simulink model "ADC"  (R2019b)
settings: Solver=FixedStepDiscrete  StartTime=0.0  StopTime=inf  FixedStep=0.05  RelTol=1e-3
libraries: discretizing x1
settings Model: Creator=Michał  LastModifiedBy=Michał
settings OptimizationCC: DefaultParameterBehavior=Inlined  EnhancedBackFolding=on  PassReuseOutputArgsAs=Individual arguments  OptimizeBlockOrder=speed  DifferentSizesBufferReuse=on  OptimizationCustomize=off  EfficientTunableParamExpr=on
settings DebuggingCC: ParameterTunabilityLossMsg=error
settings SFSimCC: MATLABDynamicMemAlloc=off
settings RTWCC: SystemTargetFile=ert.tlc  TemplateMakefile=ert_default_tmf  GenerateReport=on  IncludeHyperlinkInReport=on  LaunchReport=on  GenerateTraceInfo=on  GenerateTraceReport=on  GenerateTraceReportSl=on  GenerateTraceReportSf=on  GenerateTraceReportEml=on
settings CodeAppCC: ForceParamTrailComments=on  IgnoreCustomStorageClasses=off  OperatorAnnotations=on  SimulinkDataObjDesc=on  SFDataObjDesc=on  InsertBlockDesc=on
settings ERTTargetCC: TargetLangStandard=C99 (ISO)  GenerateSampleERTMain=on  MultiInstanceERTCode=on  CodeInterfacePackaging=Reusable function  SupportComplex=off  InlinedParameterPlacement=NonHierarchical  ERTCustomFileTemplate=example_file_process.tlc

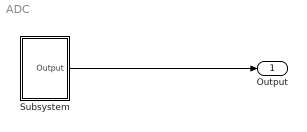
== system ADC ==
  Subsystem : Subsystem
  Output : Outport
  wires:
  Subsystem/1(Output) -> Output/1

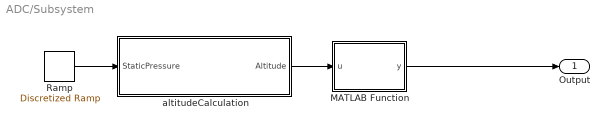
== system ADC/Subsystem ==
  MATLAB Function : MATLAB Function  TreatAsAtomicUnit=on
  Ramp : discretizing/Discretized Ramp  slope=100  start=0  X0=0  SampleTime=0.05
      settings: SourceProductName=Simulink  SourceProductBaseCode=SL
  altitudeCalculation : MATLAB Function  TreatAsAtomicUnit=on
  Output : Outport
  wires:
  altitudeCalculation/1(Altitude) -> MATLAB Function/1(u)
  Ramp/1 -> altitudeCalculation/1(StaticPressure)
  MATLAB Function/1(y) -> Output/1

== matlab function ADC/Subsystem/MATLAB Function ==
  data: u input; y output
function y = fcn(u)
if(u<100)
    y = 0;
else
    y=1;
end

== matlab function ADC/Subsystem/altitudeCalculation ==
  data: StaticPressure input; Altitude output
function Altitude  = fcn(StaticPressure)

Altitude = 44300*(1-((StaticPressure/101325)^(1/5.256)));

end
